simulink model "Inverted_Pendulum_simul"  (R2022a)
settings: Solver=VariableStepAuto  StartTime=0.0  StopTime=5  RelTol=1e-3
values from neighbouring files (symbols this model uses):
  F = [0     1      0    0 ... (first row only)    [Inverted_Pendulum.m]
  G = [   0 ... (first row only)    [Inverted_Pendulum.m]
  H = [1 0 0 0 ... (first row only)    [Inverted_Pendulum.m]
  K = acker(F,G,[s1 s2 s3 s4])    [Inverted_Pendulum.m]
  K_Integral = [K_temp_I(2) K_temp_I(3) K_temp_I(4) K_temp_I(5)]    [Inverted_Pendulum.m]
  K_Integral_SRLX = [K_temp_I_SRLX(2) K_temp_I_SRLX(3) K_temp_I_SRLX(4) K_temp_I_SRLX(5)]    [Inverted_Pendulum.m]
  K_LQR = acker(F,G,LQR_pole)    [Inverted_Pendulum.m]
  KI_integral = K_temp_I(1)    [Inverted_Pendulum.m]
  KI_integral_SRLX = K_temp_I_SRLX(1)    [Inverted_Pendulum.m]
  L = place(F',H',p_e)'    [Inverted_Pendulum.m]
  L_LQR = place(F',H',p_e_LQR)'    [Inverted_Pendulum.m]
  Nbar = Nu + K * Nx    [Inverted_Pendulum.m]
  Nbar_LQR = Nu + K_LQR * Nx    [Inverted_Pendulum.m]
  ref = 5    [Inverted_Pendulum.m]
libraries: simulink x3
settings Model: Creator=OS  LastModifiedBy=OS

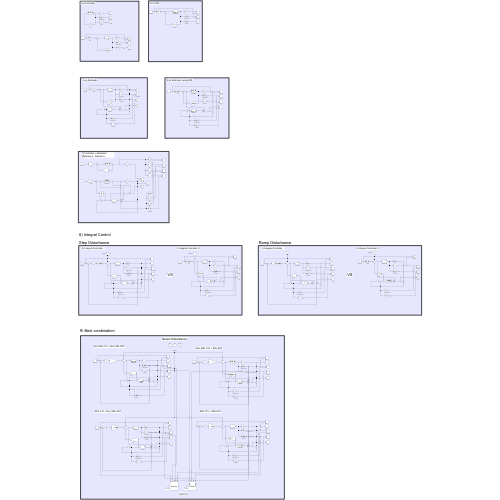
[thumbnail: Simulink's stored preview of the top-level diagram]
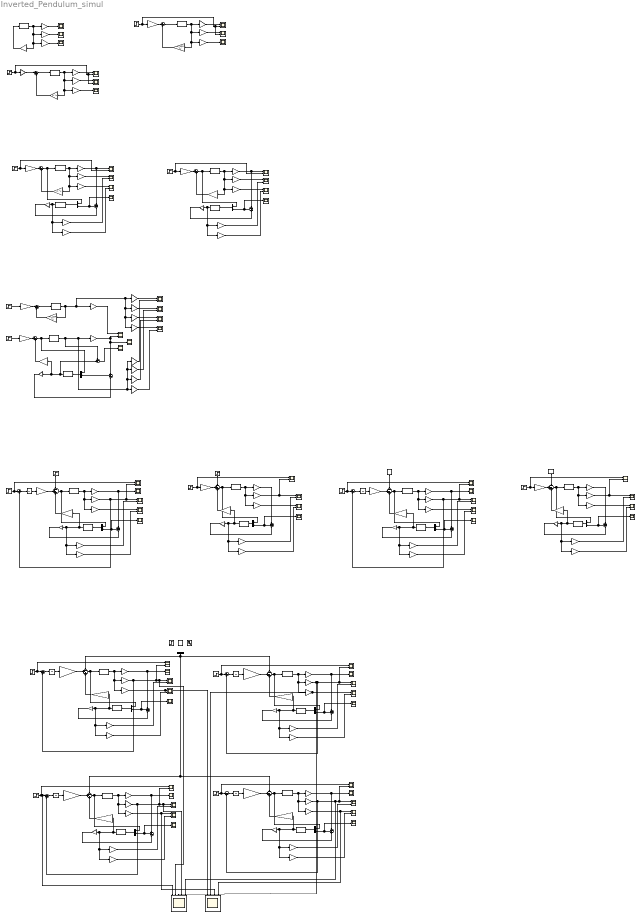
== system Inverted_Pendulum_simul ==
  note: 위치
  note: OUTPUT
  note: Select Disturbance
  note: Non SRL CTL + Non SRL EST
  note: 8) Integral Control
  note: Step Disturbance
  note: X Integral Controller X
  note: VS
  note: 6-a) Estimator
  note: 5-b) LQR
  note: 5-a) Controller
  note: 6-b) Estimator using SRL
  note: 7) Controller + Estimator (Reference - Nonzero)
  note: 8) Integral Controller
  note: X Integral Controller X
  note: Ramp Disturbance
  note: VS
  note: 8) Integral Controller
  note: 9) Best combination
  note: Non SRL CTL + SRL EST
  note: SRL CTL + Non SRL EST
  note: SRL CTL + SRL EST
  note: 각도
  " State-Space" : StateSpace  A=F  B=G  C=eye(4)  D=zeros(4,1)  InitialCondition=[0 0 10 0]  ParameterTunability=Optimized
   State-Space{1..5,7..14} (13 alike) : StateSpace  A=F  B=G  C=eye(4)  D=zeros(4,1)  InitialCondition=[0 0 0 0]  ParameterTunability=Optimized
  " State-Space6" : StateSpace  A=F  B=G  C=eye(4)  D=zeros(4,1)  InitialCondition=[0.005 0 0 0]  ParameterTunability=Optimized
  Disturbance : Step  Time=1.5  After=10  SampleTime=0
  Disturbance1 : Step  Time=1.5  After=10  SampleTime=0
  Disturbance2 : simulink/Sources/Ramp  slope=1  start=1.5  InitialOutput=0
  Disturbance3 : simulink/Sources/Ramp  slope=1  start=1.5  InitialOutput=0
  Estimator : StateSpace  A=F  B=[G L]  C=eye(4)  D=zeros(4,3)  InitialCondition=[5 0 1 0]
  Estimator1 : StateSpace  A=F  B=[G L_LQR]  C=eye(4)  D=zeros(4,3)  InitialCondition=[5 0 1 0]
  Estimator10 : StateSpace  A=F  B=[G L]  C=eye(4)  D=zeros(4,3)  InitialCondition=[0.001 0 0 0]
  Estimator2 : StateSpace  A=F  B=[G L_LQR]  C=eye(4)  D=zeros(4,3)  InitialCondition=[0 0 0 0]
  Estimator{3..6} (4 alike) : StateSpace  A=F  B=[G L_LQR]  C=eye(4)  D=zeros(4,3)  InitialCondition=[0.01 0 0 0]
  Estimator7 : StateSpace  A=F  B=[G L]  C=eye(4)  D=zeros(4,3)  InitialCondition=[0.001 0 0 0]
  Estimator8 : StateSpace  A=F  B=[G L_LQR]  C=eye(4)  D=zeros(4,3)  InitialCondition=[0.001 0 0 0]
  Estimator9 : StateSpace  A=F  B=[G L_LQR]  C=eye(4)  D=zeros(4,3)  InitialCondition=[0.001 0 0 0]
  Gain{,1..4,6..7,9..10,12,14,16} (12 alike) : Gain  Gain=H  Multiplication=Matrix(K*u)
  Gain11 : Gain  Gain=-KI_integral_SRLX
  Gain13 : Gain  Gain=-KI_integral_SRLX
  Gain{5,8,15,17} (4 alike) : Gain  Gain=-KI_integral
  Integrator{,1..5} (6 alike) : Integrator
  Mux{,1..10} (11 alike) : Mux  Inputs=2
  Mux11 : Mux  Inputs=1
  Nbar : Gain  Gain=Nbar
  Nbar{1,3..7} (6 alike) : Gain  Gain=Nbar_LQR
  Nbar2 : Gain  Gain=Nbar
  "Ramp " : simulink/Sources/Ramp  slope=5  start=1  InitialOutput=0
  Reference{,1..13} (14 alike) : Step  Time=0  After=ref  SampleTime=0
  "Sine Wave " : Sin  Amplitude=3  Frequency=10  SampleTime=0
  "Step " : Step  After=5  SampleTime=0
  Sum{,1..2,4,6..7} (6 alike) : Sum  Inputs=|++
  Sum{10,13,15,18,20,23,26,29} (8 alike) : Sum  Inputs=-|+|+
  Sum{3,5,8,11,14,16,19,21,24,27,30} (11 alike) : Sum  Inputs=+|-
  Sum{12,17,22,25,28,31} (6 alike) : Sum  Inputs=|-+
  Sum9 : Sum  Inputs=+-|
  angle : Scope
  angle1 : Scope
  angle{3..12} (10 alike) : Scope  NumInputPorts=2
  angle2 : Scope
  cart dot x : Scope  NumInputPorts=2
  cart position : Scope
  cart position{1..12} (12 alike) : Scope  NumInputPorts=2
  cart x : Scope  NumInputPorts=2
  dot theta : Gain  Gain=[0 0 0 1]  Multiplication=Matrix(K*u)
  dot theta1 : Gain  Gain=[0 0 0 1]  Multiplication=Matrix(K*u)
  dot x : Gain  Gain=[0 1 0 0]  Multiplication=Matrix(K*u)
  dot x1 : Gain  Gain=[0 1 0 0]  Multiplication=Matrix(K*u)
  error{,1..10} (11 alike) : Scope
  for angle{,1..22} (23 alike) : Gain  Gain=[0 0 1 0]  Multiplication=Matrix(K*u)
  for cart position{,1..22} (23 alike) : Gain  Gain=[1 0 0 0]  Multiplication=Matrix(K*u)
  output{,7..8,11,14,16,18,20} (8 alike) : Scope
  output{1..6,9..10,12..13,15,17,19} (13 alike) : Scope  NumInputPorts=2
  pendulum dot theta : Scope  NumInputPorts=2
  pendulum theta : Scope  NumInputPorts=2
  theta : Gain  Gain=[0 0 1 0]  Multiplication=Matrix(K*u)
  theta1 : Gain  Gain=[0 0 1 0]  Multiplication=Matrix(K*u)
  u=-K_LQR x : Gain  Gain=-K_LQR  Multiplication=Matrix(K*u)
  u=-K_LQR x1 : Gain  Gain=-K_LQR  Multiplication=Matrix(K*u)
  u=-Kx : Gain  Gain=-K  Multiplication=Matrix(K*u)
  u=-Kx1 : Gain  Gain=-K  Multiplication=Matrix(K*u)
  u=-Kx10 : Gain  Gain=-K_Integral_SRLX  Multiplication=Matrix(K*u)
  u=-Kx{5,7,11..12} (4 alike) : Gain  Gain=-K_Integral  Multiplication=Matrix(K*u)
  u=-Kx2 : Gain  Gain=-K  Multiplication=Matrix(K*u)
  u=-Kx{3..4,6,8} (4 alike) : Gain  Gain=-K_LQR  Multiplication=Matrix(K*u)
  u=-Kx9 : Gain  Gain=-K_Integral_SRLX  Multiplication=Matrix(K*u)
  x : Gain  Gain=[1 0 0 0]  Multiplication=Matrix(K*u)
  x1 : Gain  Gain=[1 0 0 0]  Multiplication=Matrix(K*u)
  y{,1..13} (14 alike) : Gain  Gain=H  Multiplication=Matrix(K*u)
  각도 : Scope  NumInputPorts=4
  위치 : Scope  NumInputPorts=5
  wires:
  u=-Kx/1 -> " State-Space"/1  "u"
  Gain1/1 -> output/1  "y"
  for angle/1 -> angle/1  "theta"
  for cart position/1 -> cart position/1  "x"
  " State-Space"/1 -> for cart position/1, u=-Kx/1, for angle/1, Gain1/1
  for cart position2/1 -> cart position2/1  "x"
  " State-Space2"/1 -> for cart position2/1, u=-Kx1/1, for angle2/1, y/1
  y/1 -> output2/1  "y"
  for angle2/1 -> angle2/1  "theta"
  u=-Kx1/1 -> Sum/2  "u"
  Sum/1 -> " State-Space2"/1
  Reference/1 -> cart position2/2, output2/2, Nbar/1
  Nbar/1 -> Sum/1
  Nbar1/1 -> Sum1/1
  Reference1/1 -> cart position1/2, output1/2, Nbar1/1
  y1/1 -> output1/1  "y"
  for angle1/1 -> angle1/1  "theta"
  for cart position1/1 -> cart position1/1  "x"
  u=-K_LQR x/1 -> Sum1/2  "u"
  Sum1/1 -> " State-Space1"/1
  " State-Space1"/1 -> for cart position1/1, u=-K_LQR x/1, for angle1/1, y1/1
  Nbar2/1 -> Sum2/1
  Reference2/1 -> output3/2, Nbar2/1
  y2/1 -> Sum3/1, output3/1  "y"
  for angle3/1 -> angle3/1  "theta"
  for cart position3/1 -> cart position3/1  "x"
  u=-Kx2/1 -> Sum2/2  "u"
  Sum2/1 -> Mux/1, " State-Space3"/1
  " State-Space3"/1 -> for cart position3/1, u=-Kx2/1, for angle3/1, y2/1
  Estimator/1 -> for angle4/1, for cart position4/1, Gain/1
  Mux/1 -> Estimator/1
  Sum3/1 -> error/1, Mux/2
  Gain/1 -> Sum3/2
  for cart position4/1 -> cart position3/2  "x"
  for angle4/1 -> angle3/2  "theta"
  y3/1 -> Sum5/1, output4/1  "y"
  u=-Kx3/1 -> Sum4/2  "u"
  Reference3/1 -> output4/2, Nbar3/1
  for cart position5/1 -> cart position4/1  "x"
  Estimator1/1 -> for angle6/1, for cart position6/1, Gain2/1
  Gain2/1 -> Sum5/2
  Sum5/1 -> error1/1, Mux1/2
  Mux1/1 -> Estimator1/1
  for cart position6/1 -> cart position4/2  "x"
  Sum4/1 -> Mux1/1, " State-Space4"/1
  for angle6/1 -> angle4/2  "theta"
  Nbar3/1 -> Sum4/1
  for angle5/1 -> angle4/1  "theta"
  " State-Space4"/1 -> for cart position5/1, u=-Kx3/1, for angle5/1, y3/1
  u=-K_LQR x1/1 -> Sum6/2  "u"
  " State-Space5"/1 -> u=-K_LQR x1/1, dot x/1, dot theta/1, theta/1, x/1, y4/1
  y4/1 -> output6/1  "y"
  Sum6/1 -> " State-Space5"/1
  Nbar4/1 -> Sum6/1
  Reference4/1 -> Nbar4/1
  y5/1 -> output7/1, Sum8/1, output6/2  "y"
  u=-Kx4/1 -> Sum7/2  "u"
  Reference5/1 -> Nbar5/1
  Estimator2/1 -> Sum9/2, Gain3/1, u=-Kx4/1
  Gain3/1 -> Sum8/2
  Sum8/1 -> Mux2/2
  Mux2/1 -> Estimator2/1
  Sum7/1 -> Mux2/1, " State-Space6"/1
  Nbar5/1 -> Sum7/1
  Sum9/1 -> error2/1
  " State-Space6"/1 -> Sum9/1, dot theta1/1, theta1/1, dot x1/1, x1/1, y5/1
  x/1 -> cart x/1
  x1/1 -> cart x/2
  dot x/1 -> cart dot x/1
  dot x1/1 -> cart dot x/2
  theta/1 -> pendulum theta/1
  theta1/1 -> pendulum theta/2
  dot theta1/1 -> pendulum dot theta/2
  dot theta/1 -> pendulum dot theta/1
  " State-Space7"/1 -> for angle7/1, for cart position7/1, y6/1
  Sum11/1 -> error3/1, Mux3/2
  for angle7/1 -> angle5/1  "theta"
  Estimator3/1 -> u=-Kx5/1, for angle8/1, for cart position8/1, Gain4/1
  Gain4/1 -> Sum11/2
  for cart position8/1 -> cart position5/2  "x"
  Mux3/1 -> Estimator3/1
  for angle8/1 -> angle5/2  "theta"
  Sum10/1 -> Mux3/1, " State-Space7"/1
  y6/1 -> output8/1, Sum11/1  "y"
  for cart position7/1 -> Sum12/2, output5/2, cart position5/1  "x"
  Reference6/1 -> output5/1, Sum12/1
  Integrator/1 -> Gain5/1
  Sum12/1 -> Integrator/1
  Gain5/1 -> Sum10/2
  u=-Kx5/1 -> Sum10/3  "u"
  Disturbance/1 -> Sum10/1
  " State-Space8"/1 -> for cart position9/1, for angle9/1, y7/1
  Sum14/1 -> error4/1, Mux4/2
  for angle9/1 -> angle6/1  "theta"
  Estimator4/1 -> u=-Kx6/1, for angle10/1, for cart position10/1, Gain6/1
  Gain6/1 -> Sum14/2
  for cart position10/1 -> cart position6/2  "x"
  Mux4/1 -> Estimator4/1
  for angle10/1 -> angle6/2  "theta"
  Sum13/1 -> Mux4/1, " State-Space8"/1
  y7/1 -> Sum14/1  "y"
  for cart position9/1 -> output9/2, cart position6/1  "x"
  Reference7/1 -> output9/1, Nbar6/1
  Nbar6/1 -> Sum13/2
  u=-Kx6/1 -> Sum13/3  "u"
  Disturbance1/1 -> Sum13/1
  u=-Kx7/1 -> Sum15/3  "u"
  Disturbance2/1 -> Sum15/1
  Sum17/1 -> Integrator1/1
  y9/1 -> Sum19/1  "y"
  Sum18/1 -> Mux6/1, " State-Space10"/1
  Gain8/1 -> Sum15/2
  for angle14/1 -> angle8/1  "theta"
  Sum19/1 -> error6/1, Mux6/2
  Mux6/1 -> Estimator6/1
  for cart position14/1 -> output12/2, cart position8/1  "x"
  Reference9/1 -> output12/1, Nbar7/1
  for cart position11/1 -> cart position8/2  "x"
  for cart position12/1 -> Sum17/2, output10/2, cart position7/1  "x"
  y8/1 -> output11/1, Sum16/1  "y"
  " State-Space10"/1 -> for cart position14/1, for angle14/1, y9/1
  Gain7/1 -> Sum16/2
  Estimator5/1 -> u=-Kx7/1, for angle13/1, for cart position13/1, Gain7/1
  Integrator1/1 -> Gain8/1
  for angle12/1 -> angle7/1  "theta"
  Gain9/1 -> Sum19/2
  Reference8/1 -> output10/1, Sum17/1
  Sum16/1 -> error5/1, Mux5/2
  " State-Space9"/1 -> for angle12/1, for cart position12/1, y8/1
  u=-Kx8/1 -> Sum18/3  "u"
  Disturbance3/1 -> Sum18/1
  Estimator6/1 -> u=-Kx8/1, for angle11/1, for cart position11/1, Gain9/1
  for cart position13/1 -> cart position7/2  "x"
  Sum15/1 -> Mux5/1, " State-Space9"/1
  for angle13/1 -> angle7/2  "theta"
  for angle11/1 -> angle8/2  "theta"
  Nbar7/1 -> Sum18/2
  Mux5/1 -> Estimator5/1
  u=-Kx9/1 -> Sum20/3  "u"
  Sum22/1 -> Integrator2/1
  Gain11/1 -> Sum20/2
  for cart position15/1 -> cart position9/1, 위치/2, output13/2, Sum22/2  "Non SRL CTL + Non SRL EST x"
  y10/1 -> output14/1, Sum21/1  "y"
  Gain10/1 -> Sum21/2
  Estimator7/1 -> u=-Kx9/1, for angle16/1, for cart position16/1, Gain10/1
  Integrator2/1 -> Gain11/1
  for angle15/1 -> 각도/1, angle9/1  "Non SRL CTL + Non SRL EST theta"
  Reference10/1 -> output13/1, Sum22/1
  " State-Space11"/1 -> for angle15/1, for cart position15/1, y10/1
  for cart position16/1 -> cart position9/2  "x"
  Sum21/1 -> error7/1, Mux7/2
  Sum20/1 -> Mux7/1, " State-Space11"/1
  for angle16/1 -> angle9/2  "theta"
  Mux7/1 -> Estimator7/1
  Mux8/1 -> Estimator8/1
  Sum24/1 -> error8/1, Mux8/2
  Sum23/1 -> Mux8/1, " State-Space12"/1
  " State-Space12"/1 -> for angle17/1, for cart position17/1, y11/1
  for cart position18/1 -> cart position10/2  "x"
  for angle18/1 -> angle10/2  "theta"
  Reference11/1 -> output15/1, Sum25/1
  Estimator8/1 -> u=-Kx10/1, for angle18/1, for cart position18/1, Gain12/1
  for angle17/1 -> angle10/1, 각도/2  "Non SRL CTL + SRL EST theta"
  y11/1 -> output16/1, Sum24/1  "y"
  Integrator3/1 -> Gain13/1
  Gain12/1 -> Sum24/2
  Sum25/1 -> Integrator3/1
  u=-Kx10/1 -> Sum23/3  "u"
  for cart position17/1 -> 위치/3, cart position10/1, output15/2, Sum25/2  "Non SRL CTL + SRL EST x"
  Gain13/1 -> Sum23/2
  Gain15/1 -> Sum26/2
  Sum28/1 -> Integrator4/1
  Gain14/1 -> Sum27/2
  Integrator4/1 -> Gain15/1
  for angle19/1 -> angle11/1, 각도/4  "SRL CTL + SRL EST theta"
  Reference12/1 -> output17/1, Sum28/1
  for angle20/1 -> angle11/2  "theta"
  Sum26/1 -> Mux9/1, " State-Space13"/1
  Estimator9/1 -> u=-Kx11/1, for angle20/1, for cart position20/1, Gain14/1
  u=-Kx11/1 -> Sum26/3  "u"
  for cart position20/1 -> cart position11/2  "x"
  Sum27/1 -> error9/1, Mux9/2
  y12/1 -> output18/1, Sum27/1  "y"
  Mux9/1 -> Estimator9/1
  for cart position19/1 -> output17/2, cart position11/1, 위치/5, Sum28/2  "SRL CTL + SRL EST x"
  " State-Space13"/1 -> for angle19/1, for cart position19/1, y12/1
  Reference13/1 -> 위치/1, Sum31/1, output19/1
  u=-Kx12/1 -> Sum29/3  "u"
  Estimator10/1 -> u=-Kx12/1, for angle22/1, for cart position22/1, Gain16/1
  " State-Space14"/1 -> for angle21/1, for cart position21/1, y13/1
  for cart position21/1 -> 위치/4, cart position12/1, output19/2, Sum31/2  "SRL CTL + Non SRL EST x"
  Integrator5/1 -> Gain17/1
  Mux10/1 -> Estimator10/1
  Sum31/1 -> Integrator5/1
  Gain17/1 -> Sum29/2
  y13/1 -> output20/1, Sum30/1  "y"
  for angle22/1 -> angle12/2  "theta"
  Gain16/1 -> Sum30/2
  for cart position22/1 -> cart position12/2  "x"
  for angle21/1 -> 각도/3, angle12/1  "SRL CTL + Non SRL EST theta"
  Sum29/1 -> Mux10/1, " State-Space14"/1
  Sum30/1 -> error10/1, Mux10/2
  Mux11/1 -> Sum20/1, Sum29/1, Sum26/1, Sum23/1
